simulink model "case_4_cut_out"  (R2025a)
settings: Solver=VariableStepAuto  StartTime=0.0  StopTime=150  RelTol=1e-3
settings Model: Creator=sanborkl  LastModifiedBy=admin

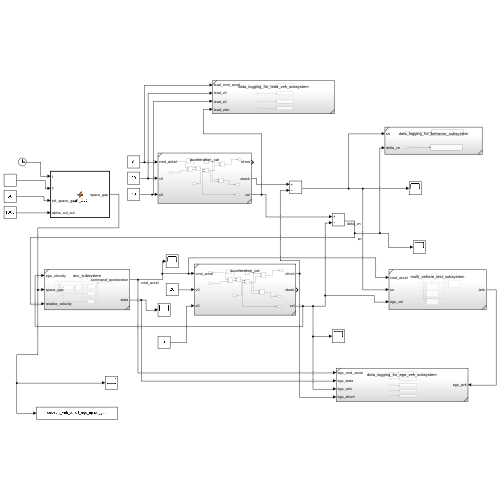
[thumbnail: Simulink's stored preview of the top-level diagram]
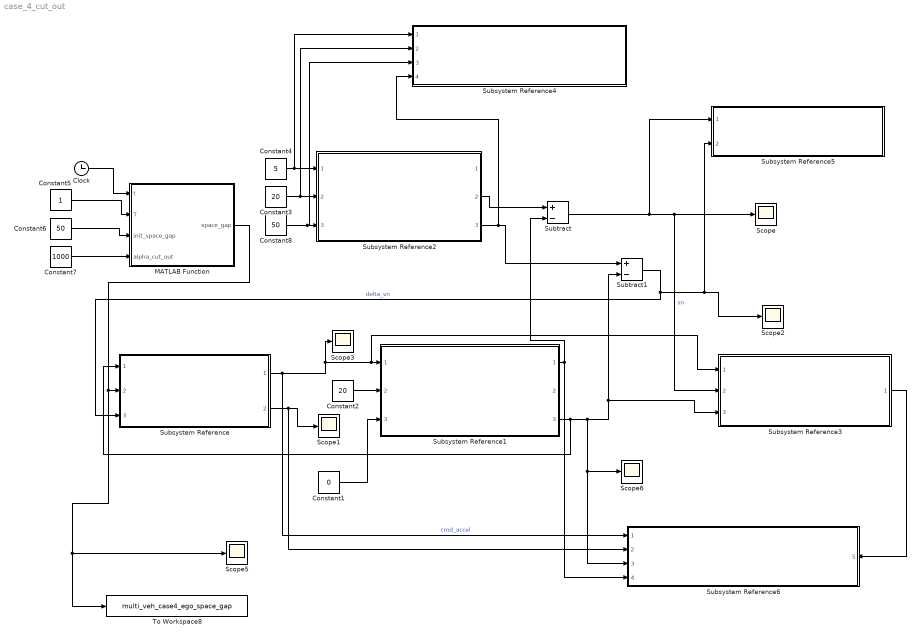
== system case_4_cut_out ==
  Clock : Clock
  Constant1 : Constant  Value=0
  Constant2 : Constant  Value=20
  Constant3 : Constant  Value=20
  Constant4 : Constant  Value=5
  Constant5 : Constant
  Constant6 : Constant  Value=50
  Constant7 : Constant  Value=1000
  Constant8 : Constant  Value=50
  MATLAB Function : MATLAB Function  TreatAsAtomicUnit=on
  Scope{,1..3,5..6} (6 alike) : Scope
      Scope settings: ActiveDisplayYMinimum=-6713.614999999998  ActiveDisplayYMaximum=60880.134999999995
      Scope1 settings: ActiveDisplayYMinimum=-1  ActiveDisplayYMaximum=1  DataLoggingVariableName=ScopeData2
      Scope2 settings: ActiveDisplayYMinimum=-91.874999999999986  ActiveDisplayYMaximum=826.875  DataLoggingVariableName=ScopeData3
      Scope3 settings: ActiveDisplayYMinimum=0.053894456452525219  ActiveDisplayYMaximum=1.9288944564525257  DataLoggingVariableName=ScopeData4
      Scope5 settings: ActiveDisplayYMinimum=-37.436177326152972  ActiveDisplayYMaximum=308.42268451722509  DataLoggingVariableName=ScopeData5
      Scope6 settings: ActiveDisplayYMinimum=18.125  ActiveDisplayYMaximum=36.875  DataLoggingVariableName=ScopeData6
  Subsystem Reference : Subsystem  ReferencedSubsystem=acc_subsystem
  Subsystem Reference1 : Subsystem  ReferencedSubsystem=acceleration_car
  Subsystem Reference2 : Subsystem  ReferencedSubsystem=acceleration_car
  Subsystem Reference3 : Subsystem  ReferencedSubsystem=multi_vehicle_test_subsystem
  Subsystem Reference4 : Subsystem  ReferencedSubsystem=data_logging_for_lead_veh_subsystem
  Subsystem Reference5 : Subsystem  ReferencedSubsystem=data_logging_for_behavior_subsystem
  Subsystem Reference6 : Subsystem  ReferencedSubsystem=data_logging_for_ego_veh_subsystem
      settings: PortSchema="{\"entries\":[{\"content\":{\"sides\":[{\"content\":{\"connectorIds\":[\"In1\",\"In2\",\"In3\",\"In4\"]},\"type\":\"ConnectorPlacement.EquallySpacedRectSide\",\"uuid\":\"1bb3a8cf-f981-4f8a-aff9-03896ccf7d7c\"},{\"content\":{\"connectorIds\":[\"In5\"],\"side\":\"RIGHT\"},\"type\":\"ConnectorPlacement.EquallySpacedRectSide\",\"uuid\":\"3f6ac5cb-96be-44a3-8993-3635a91bd658\"},{\"content\":{\"side\":\"TOP\"},\"type\":\"ConnectorPlacement.EquallySpacedRectSide\",\"uuid\":\"c641fc7f-a424-4033-b273-2526f6b205c0\"}]},\"type\":\"ConnectorPlacement.EquallySpacedConnector\",\"uuid\":\"2a4be48e-084e-4aa6-b74f-8fe234fedc1a\"}],\"packageUris\":[\"http://schema.mathworks.com/mf0/Connector/R2020b\"],\"version\":\"1.0\"}"
  Subtract : Sum  Inputs=+-
  Subtract1 : Sum  Inputs=+-
  To Workspace8 : ToWorkspace  VariableName=multi_veh_case4_ego_space_gap  SaveFormat=Structure With Time  SampleTime=-1
  wires:
  Constant2/1 -> Subsystem Reference1/2
  Constant1/1 -> Subsystem Reference1/3
  Subsystem Reference2/2 -> Subtract/1
  Subtract/1 -> Subsystem Reference5/1, Subsystem Reference3/2, Scope/1  "sn"
  Subtract1/1 -> Subsystem Reference5/2, Scope2/1, Subsystem Reference/3  "delta_vn"
  Clock/1 -> MATLAB Function/1(t)
  Constant5/1 -> MATLAB Function/2(T)
  Constant6/1 -> MATLAB Function/3(init_space_gap)
  Constant7/1 -> MATLAB Function/4(alpha_cut_out)
  MATLAB Function/1(space_gap) -> To Workspace8/1, Scope5/1, Subsystem Reference/2
  Constant4/1 -> Subsystem Reference4/1, Subsystem Reference2/1
  Constant3/1 -> Subsystem Reference4/2, Subsystem Reference2/2
  Constant8/1 -> Subsystem Reference4/3, Subsystem Reference2/3
  Subsystem Reference2/3 -> Subsystem Reference4/4, Subtract1/1
  Subsystem Reference1/1 -> Subtract/2, Subsystem Reference6/4
  Subsystem Reference/1 -> Subsystem Reference6/1, Scope3/1, Subsystem Reference3/1, Subsystem Reference1/1  "cmd_accel"
  Subsystem Reference/2 -> Subsystem Reference6/2, Scope1/1
  Subsystem Reference3/1 -> Subsystem Reference6/5
  Subsystem Reference1/3 -> Subsystem Reference/1, Subsystem Reference6/3, Scope6/1, Subtract1/2, Subsystem Reference3/3

== matlab function case_4_cut_out/MATLAB Function ==
  data: t input; space_gap output; T input; init_space_gap input; alpha_cut_out input
function space_gap = cut_out(t, T, init_space_gap , alpha_cut_out)

% alpha_cut_out is how fast the lead car is getting out, 
% for this case, alpha_cut_out is low

if t < T
    space_gap = init_space_gap;
else
    space_gap = min(init_space_gap + t * alpha_cut_out, 255);
end
